simulink model "SysModel"  (R2018a)
settings: Solver=ode5  StartTime=0.0  StopTime=10  FixedStep=1e-3  MaxStep=0.01  RelTol=1e-4  EnableMultiTasking=on
libraries: simulink x2
settings Model: Creator=Risky Jr  LastModifiedBy=Risky Jr
settings DataIOCC: LimitDataPoints=on  SaveOutput=off  SaveTime=off
settings OptimizationCC: ExpressionDepthLimit=2147483647  LifeSpan=1
settings DebuggingCC: UnderspecifiedInitializationDetection=Classic  MergeDetectMultiDrivingBlocksExec=none  FcnCallInpInsideContextMsg=warning  AllowSymbolicDim=off  StateNameClashWarn=warning  SFUnexpectedBacktrackingDiag=warning  SFNoUnconditionalDefaultTransitionDiag=warning  SFExecutionAtInitializationDiag=none
settings CodeAppCC: StateflowObjectComments=on
settings GRTTargetCC: TargetLangStandard=C89/C90 (ANSI)  GeneratePreprocessorConditionals=Disable all  CombineOutputUpdateFcns=off  GRTInterface=on

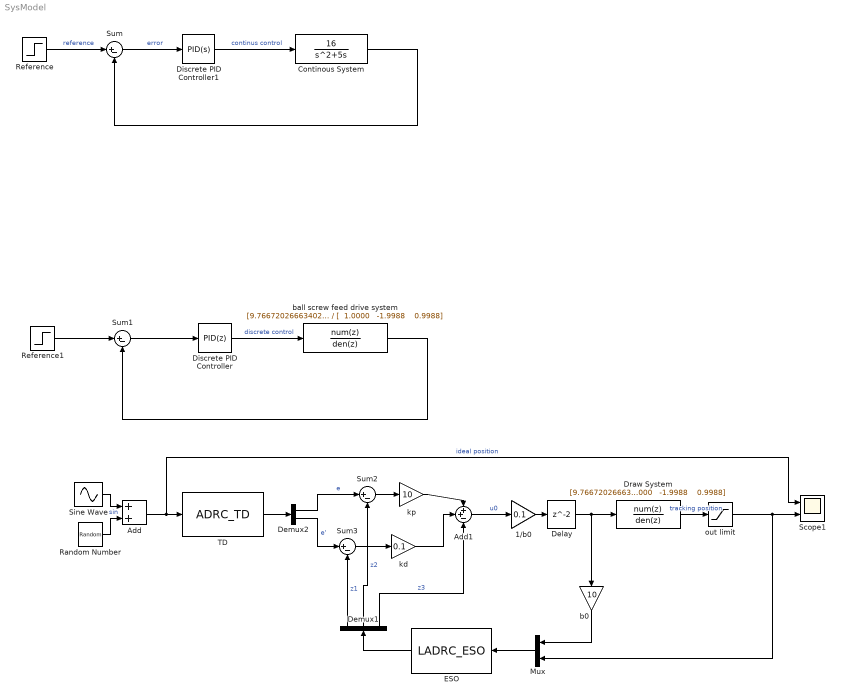
== system SysModel ==
  " ball screw feed drive system" : DiscreteTransferFcn  Numerator=[9.766720266634020e-07 1.841743524655902e-06 8.650714979924997e-07]  Denominator="[  1.0000   -1.9988    0.9988]"  SampleTime=1e-3
  1/b0 : Gain  Gain=0.1
  Add : Sum
  Add1 : Sum  Inputs=++-
  Continous System : TransferFcn  Numerator=[16]  Denominator=[1 5 0]
  Delay : Delay
  Demux1 : Demux  Outputs=3
  Demux2 : Demux  Outputs=2
  Discrete PID Controller : simulink/Continuous/PID Controller  Controller=PID  TimeDomain=Discrete-time  SampleTime=1e-3  IntegratorMethod=Forward Euler  FilterMethod=Forward Euler  Form=Parallel  UseFilter=on  ControllerParametersSource=internal  P=1  I=0  D=0  N=100  InitialConditionSource=internal  InitialConditionForIntegrator=0  InitialConditionForFilter=0  ExternalReset=none  LimitOutput=off  UpperSaturationLimit=inf  LowerSaturationLimit=-inf  LinearizeAsGain=off  AntiWindupMode=none  Kb=1  TrackingMode=off  Kt=1  PParamMin=[]  PParamMax=[]  IParamMin=[]  IParamMax=[]  DParamMin=[]  DParamMax=[]  NParamMin=[]  NParamMax=[]  KbParamMin=[]  KbParamMax=[]  KtParamMin=[]  KtParamMax=[]  POutMin=[]  POutMax=[]  IOutMin=[]  IOutMax=[]  DOutMin=[]  DOutMax=[]  NOutMin=[]  NOutMax=[]  KbOutMin=[]  KbOutMax=[]  KtOutMin=[]  KtOutMax=[]  IntegratorOutMin=[]  IntegratorOutMax=[]  FilterOutMin=[]  FilterOutMax=[]  SumOutMin=[]  SumOutMax=[]  SumI1OutMin=[]  SumI1OutMax=[]  SumI2OutMin=[]  SumI2OutMax=[]  SumI3OutMin=[]  SumI3OutMax=[]  SumDOutMin=[]  SumDOutMax=[]  SaturationOutMin=[]  SaturationOutMax=[]  IntegratorContinuousStateAttributes=''  IntegratorStateMustResolveToSignalObject=off  IntegratorRTWStateStorageClass=Auto  FilterContinuousStateAttributes=''  FilterStateMustResolveToSignalObject=off  FilterRTWStateStorageClass=Auto  DifferentiatorICPrevScaledInput=0  DifferentiatorOutMin=[]  DifferentiatorOutMax=[]  FilterDiffOutCoefMin=[]  FilterDiffOutCoefMax=[]  SumDenOutMin=[]  SumDenOutMax=[]  SumNumOutMin=[]  SumNumOutMax=[]  ReciprocalOutMin=[]  ReciprocalOutMax=[]  DivideOutMin=[]  DivideOutMax=[]  TunerSelectOption=Transfer Function Based (PID Tuner App)
  Discrete PID Controller1 : simulink/Continuous/PID Controller  Controller=PID  TimeDomain=Continuous-time  SampleTime=-1  IntegratorMethod=Forward Euler  FilterMethod=Forward Euler  Form=Parallel  UseFilter=on  ControllerParametersSource=internal  P=1  I=0  D=0  N=100  InitialConditionSource=internal  InitialConditionForIntegrator=0  InitialConditionForFilter=0  ExternalReset=none  LimitOutput=off  UpperSaturationLimit=inf  LowerSaturationLimit=-inf  LinearizeAsGain=off  AntiWindupMode=none  Kb=1  TrackingMode=off  Kt=1  PParamMin=[]  PParamMax=[]  IParamMin=[]  IParamMax=[]  DParamMin=[]  DParamMax=[]  NParamMin=[]  NParamMax=[]  KbParamMin=[]  KbParamMax=[]  KtParamMin=[]  KtParamMax=[]  POutMin=[]  POutMax=[]  IOutMin=[]  IOutMax=[]  DOutMin=[]  DOutMax=[]  NOutMin=[]  NOutMax=[]  KbOutMin=[]  KbOutMax=[]  KtOutMin=[]  KtOutMax=[]  IntegratorOutMin=[]  IntegratorOutMax=[]  FilterOutMin=[]  FilterOutMax=[]  SumOutMin=[]  SumOutMax=[]  SumI1OutMin=[]  SumI1OutMax=[]  SumI2OutMin=[]  SumI2OutMax=[]  SumI3OutMin=[]  SumI3OutMax=[]  SumDOutMin=[]  SumDOutMax=[]  SaturationOutMin=[]  SaturationOutMax=[]  IntegratorContinuousStateAttributes=''  IntegratorStateMustResolveToSignalObject=off  IntegratorRTWStateStorageClass=Auto  FilterContinuousStateAttributes=''  FilterStateMustResolveToSignalObject=off  FilterRTWStateStorageClass=Auto  DifferentiatorICPrevScaledInput=0  DifferentiatorOutMin=[]  DifferentiatorOutMax=[]  FilterDiffOutCoefMin=[]  FilterDiffOutCoefMax=[]  SumDenOutMin=[]  SumDenOutMax=[]  SumNumOutMin=[]  SumNumOutMax=[]  ReciprocalOutMin=[]  ReciprocalOutMax=[]  DivideOutMin=[]  DivideOutMax=[]  TunerSelectOption=Transfer Function Based (PID Tuner App)
  "Draw System " : DiscreteTransferFcn  Numerator=[9.766720266634020e-07 1.841743524655902e-06 8.650714979924997e-07]  Denominator="[  1.0000   -1.9988    0.9988]"  SampleTime=1e-3
  "ESO " : S-Function  FunctionName=LADRC_ESO  Parameters=10,10,300,1000  SFunctionDeploymentMode=off  EnableBusSupport=off
  Mux : Mux  Inputs=2
  Random Number : RandomNumber  Variance=0.001  SampleTime=0.001
  Reference : Step  SampleTime=0
  Reference1 : Step  SampleTime=1e-3
  Scope1 : Scope  NumInputPorts=2
  Sine Wave : Sin  Frequency=62.8  SampleTime=1e-3
  Sum{,1..3} (4 alike) : Sum  Inputs=|+-
  TD : S-Function  FunctionName=ADRC_TD  Parameters=5,1e4  SFunctionDeploymentMode=off  EnableBusSupport=off
  b0 : Gain  Gain=10
  kd : Gain  Gain=0.1
  kp : Gain  Gain=10
  "out limit " : Saturate
  wires:
  Reference/1 -> Sum/1  "reference"
  Continous System/1 -> Sum/2
  Sum/1 -> Discrete PID Controller1/1  "error"
  Discrete PID Controller1/1 -> Continous System/1  "continus control"
  " ball screw feed drive system"/1 -> Sum1/2
  Reference1/1 -> Sum1/1
  Sum1/1 -> Discrete PID Controller/1
  Discrete PID Controller/1 -> " ball screw feed drive system"/1  "discrete control"
  Sine Wave/1 -> Add/1  "sin"
  Add/1 -> Scope1/1, TD/1  "ideal position"
  Random Number/1 -> Add/2
  "ESO "/1 -> Demux1/1
  TD/1 -> Demux2/1
  kp/1 -> Add1/1
  kd/1 -> Add1/2
  Add1/1 -> 1/b0/1  "u0"
  Mux/1 -> "ESO "/1
  "Draw System "/1 -> "out limit "/1  "tracking position"
  Demux1/3 -> Add1/3  "z3"
  Sum2/1 -> kp/1
  Demux1/2 -> Sum2/2  "z2"
  Demux2/1 -> Sum2/1  "e"
  Demux2/2 -> Sum3/1  "e'"
  Demux1/1 -> Sum3/2  "z1"
  Sum3/1 -> kd/1
  Delay/1 -> b0/1, "Draw System "/1
  1/b0/1 -> Delay/1
  b0/1 -> Mux/1
  "out limit "/1 -> Scope1/2, Mux/2
